simulink model "Maschinenmodell"  (R2013a)
settings: Solver=ode45  StartTime=0.0  StopTime=10.0  RelTol=1e-3
values from neighbouring files (symbols this model uses):
  p = 4    [parameter.mat]
undefined symbols (not defined in the file or in its folder): Jmech, Ls, Psi, Rs
settings Model: Creator=Jan  LastModifiedBy=Jan

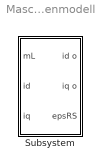
== system Maschinenmodell ==
  Subsystem : Subsystem

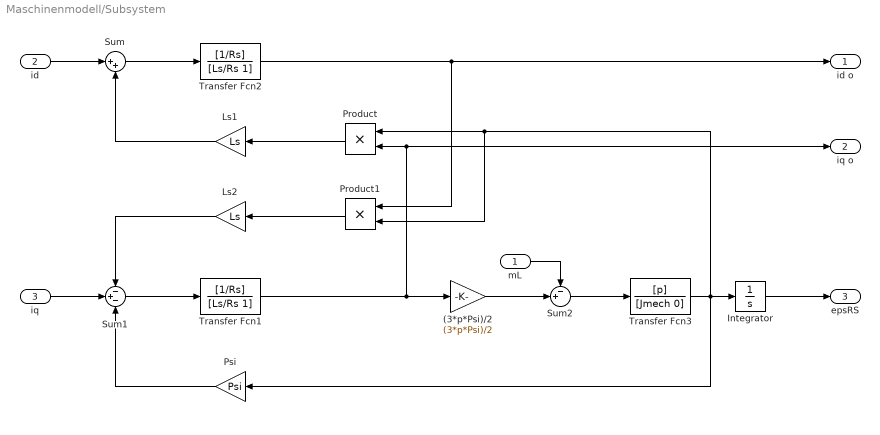
== system Maschinenmodell/Subsystem ==
  mL : Inport
  id : Inport  Port=2
  iq : Inport  Port=3
  (3*p*Psi)/2 : Gain  Gain=(3*p*Psi)/2
  Integrator : Integrator
  Ls1 : Gain  Gain=Ls
  Ls2 : Gain  Gain=Ls
  Product : Product  RndMeth=Zero
  Product1 : Product  RndMeth=Zero
  Psi : Gain  Gain=Psi
  Sum : Sum  Inputs=|++
  Sum1 : Sum  Inputs=-+-
  Sum2 : Sum  Inputs=-+|
  Transfer Fcn1 : TransferFcn  Numerator=[1/Rs]  Denominator=[Ls/Rs 1]
  Transfer Fcn2 : TransferFcn  Numerator=[1/Rs]  Denominator=[Ls/Rs 1]
  Transfer Fcn3 : TransferFcn  Numerator=[p]  Denominator=[Jmech 0]
  id o : Outport
  iq o : Outport  Port=2
  epsRS : Outport  Port=3
  wires:
  Product/1 -> Ls1/1
  Ls2/1 -> Sum1/1
  Product1/1 -> Ls2/1
  Sum1/1 -> Transfer Fcn1/1
  Sum/1 -> Transfer Fcn2/1
  Ls1/1 -> Sum/2
  Integrator/1 -> epsRS/1
  (3*p*Psi)/2/1 -> Sum2/2
  Psi/1 -> Sum1/3
  id/1 -> Sum/1
  mL/1 -> Sum2/1
  iq/1 -> Sum1/2
  Transfer Fcn2/1 -> id o/1, Product1/1
  Sum2/1 -> Transfer Fcn3/1
  Transfer Fcn3/1 -> Psi/1, Product1/2, Product/1, Integrator/1
  Transfer Fcn1/1 -> iq o/1, Product/2, (3*p*Psi)/2/1
